simulink model "ESC_fun"  (R2020b)
settings: Solver=VariableStepAuto  StartTime=0.0  StopTime=300  RelTol=1e-3
libraries: simulink_extras x1
settings Model: Creator=Calle  LastModifiedBy=Calle

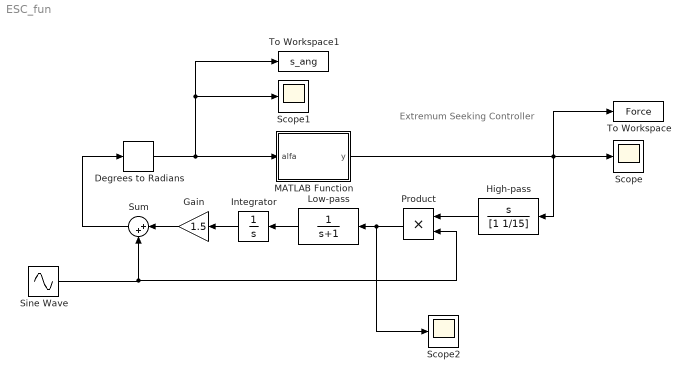
== system ESC_fun ==
  note: Extremum Seeking Controller
  Degrees to Radians : simulink_extras/Transformations/Degrees to Radians
  Gain : Gain  Gain=1.5
  High-pass : TransferFcn  Numerator=[1 0]  Denominator=[1 1/15]
  Integrator : Integrator
  Low-pass : TransferFcn  Denominator=[1 1]
  MATLAB Function : MATLAB Function  TreatAsAtomicUnit=on
  Product : Product
  Scope : Scope
  Scope1 : Scope
  Scope2 : Scope
  Sine Wave : Sin  Frequency=1/10*2*pi  SampleTime=0
  Sum : Sum  Inputs=|++
  To Workspace : ToWorkspace  VariableName=Force  SaveFormat=Timeseries  SampleTime=-1
  To Workspace1 : ToWorkspace  VariableName=s_ang  SaveFormat=Timeseries  SampleTime=-1
  wires:
  Gain/1 -> Sum/1
  Integrator/1 -> Gain/1
  Product/1 -> Low-pass/1, Scope2/1
  High-pass/1 -> Product/1
  Sine Wave/1 -> Product/2, Sum/2
  Degrees to Radians/1 -> To Workspace1/1, Scope1/1, MATLAB Function/1(alfa)
  Sum/1 -> Degrees to Radians/1
  MATLAB Function/1(y) -> Scope/1, High-pass/1, To Workspace/1
  Low-pass/1 -> Integrator/1

== matlab function ESC_fun/MATLAB Function ==
  data: alfa input; y output
function y = fcn(alfa)

    % alfa,cl,cd cm
    clcdcm = [0   0     0.0026    0
    1.0000    0.0996    0.0039    0
    2.0000    0.2010    0.0052    0
    3.0000    0.3039    0.0066    0
    4.0000    0.4083    0.0080    0
    5.0000    0.5141    0.0094    0
    6.0000    0.6252    0.0109    0.0000
    7.0000    0.7371    0.0123    0.0100
    8.0000    0.8397    0.0138    0.0150
    9.0000    0.9320    0.0154    0.0150
    10.0000    1.0188    0.0174    0.0300
    11.0000    1.1045    0.0197    0.0320
    12.0000    1.1827    0.0221    0.0330
    13.0000    1.2499    0.0248    0.0350
    14.0000    1.2946    0.0282    0.0400
    15.0000    1.3045    0.0322    0.0500
    16.0000    1.3101    0.0373    0.0200
    17.0000    1.3118    0.0435    0.0150
    18.0000    1.3119    0.0513    0.0100
    19.0000    1.3119    0.0680    0.0050
    20.0000    1.3119    0.1000         0
    21.0000    1.2969    0.2256   -0.0250
    22.0000    1.2647    0.3135   -0.0500
    23.0000    1.2130    0.3613   -0.0533
    24.0000    1.1530    0.3988   -0.0567
    25.0000    1.0971    0.4292   -0.0600
    26.0000    1.0394    0.4555   -0.0760
    27.0000    0.9732    0.4812   -0.0920
    28.0000    0.9151    0.5092   -0.1080
    29.0000    0.8795    0.5425   -0.1240
    30.0000    0.8699    0.5777   -0.1400
    35.0000    0.9667    0.7549   -0.1500
    40.0000    1.0380    0.9162   -0.1600
    45.0000    1.0503    1.0657   -0.1600
    50.0000    1.0267    1.2064   -0.2600
    55.0000    0.9744    1.3410   -0.0500
    60.0000    0.8908    1.4705   -0.2700
    65.0000    0.7665    1.5773   -0.1500
    70.0000    0.6417    1.6660   -0.4000
    75.0000    0.5126    1.7387   -0.3000
    80.0000    0.3763    1.7814   -0.2000
    85.0000    0.2367    1.7998   -0.4000
    90.0000    0.0961    1.8043   -0.4500
    95.0000   -0.0431    1.7906   -0.4200
    100.0000   -0.1820    1.7642   -0.4500
    105.0000   -0.3167    1.7114   -0.4500
    110.0000   -0.4421    1.6471   -0.2000
    115.0000   -0.5591    1.5679   -0.4000
    120.0000   -0.6714    1.4745   -0.5500
    125.0000   -0.7695    1.3653   -0.5000
    130.0000   -0.8413    1.2408   -0.5000
    135.0000   -0.9382    1.0995   -0.5400
    140.0000   -0.9777    0.9406   -0.4700
    145.0000   -0.9165    0.7655   -0.4000
    150.0000   -0.7731    0.5921   -0.4000
    155.0000   -0.6644    0.4428   -0.3200
    160.0000   -0.6400    0.3323   -0.3000
    165.0000   -0.6805    0.2363   -0.3500
    170.0000   -0.8460    0.1533   -0.4200
    175.0000   -0.6705    0.0648   -0.3000
    180.0000         0    0.0311         0];

    tmp = interp1(clcdcm(:,1),clcdcm(:,2:4),abs(rad2deg(alfa)),'pchip');
    cl = tmp(:,1).*sign(alfa)';
    cd = tmp(:,2);
    cm = tmp(:,3);

    rho = 1.225; % kg/m^3
    v = 5; % m/s
    
    h1 = 1333.33/1000; %[m] höjd för del 1
    c1 = (878.25+807.29)/2000; %[m]Korda för del 1
    h2 = 666.67/1000; %[m] höjd för del 2
    c2 = (757.11+640.50)/2000; %[m] Korda för del 2
    h3 = 666.67/1000; %[m] höjd för del 3
    c3 = (586.67+319.8)/2000; %[m] Korda för del 3
  
    %Lift - minus för att få rätt riktning
    L1 = -1/2*rho*v^2*c1*h1*cl;
    L2 = -1/2*rho*v^2*c2*h2*cl;
    L3 = -1/2*rho*v^2*c3*h3*cl;
    L = L1 + L2 + L3; %minus för att få rätt riktning

    %Drag - minus för att få rätt riktning
    D1 = -1/2*rho*v^2*c1*h1*cd;
    D2 = -1/2*rho*v^2*c2*h2*cd;
    D3 = -1/2*rho*v^2*c3*h3*cd;
    D = D1 + D2 + D3;

    Fx = D.*cos(alfa) - L.*sin(alfa);
    Fy = D.*sin(alfa) + L.*cos(alfa);

y = Fx;
